simulink model "MCC_FUZZY"  (R2024a)
settings: Solver=VariableStepAuto  StartTime=0.0  StopTime=100.0  RelTol=1e-3
model workspace (MAT data in the model file):
  J = Simulink.Parameter
  J.Complexity = 'real'
  J.Dimensions = [0 0]
  J.DataType = 'auto'
  K = Simulink.Parameter
  K.Complexity = 'real'
  K.Dimensions = [0 0]
  K.DataType = 'auto'
  Kh = Simulink.Parameter
  Kh.Complexity = 'real'
  Kh.Dimensions = [0 0]
  Kh.DataType = 'auto'
  L = Simulink.Parameter
  L.Complexity = 'real'
  L.Dimensions = [0 0]
  L.DataType = 'auto'
  R = Simulink.Parameter
  R.Complexity = 'real'
  R.Dimensions = [0 0]
  R.DataType = 'auto'
  f = Simulink.Parameter
  f.Complexity = 'real'
  f.Dimensions = [0 0]
  f.DataType = 'auto'
libraries: fuzblock x1
settings Model: Creator=NB  LastModifiedBy=NB

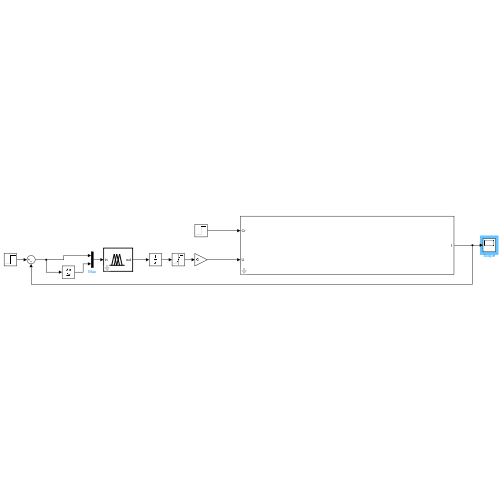
[thumbnail: Simulink's stored preview of the top-level diagram]
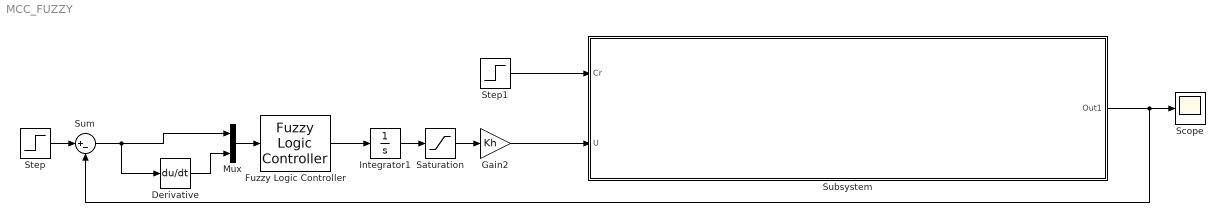
== system MCC_FUZZY ==
  Derivative : Derivative
  Fuzzy Logic Controller : fuzblock/Fuzzy Logic  Controller  FIS=FuzzyMCC  OutputSampleNumber=101  DataType=double  FuzzifiedInputs=off  RuleFiringStrengths=off  RuleOutputs=off  AggregatedOutputs=off  SimulateUsing=Interpreted execution  OutOfRangeInputValueMessage=warning  NoRuleFiredMessage=warning  EmptyOutputFuzzySetMessage=warning
  Gain2 : Gain  Gain=Kh  mask{Kh=1}
      mask prompts: Kh "entre Kh"
  Integrator1 : Integrator
  Mux : Mux  Inputs=2
  Saturation : Saturate  UpperLimit=220  LowerLimit=0
  Scope : Scope
  Step : Step  Time=0  After=100  SampleTime=0
  Step1 : Step  Time=50  After=0.05  SampleTime=0
  Subsystem : Subsystem  mask{R=2, L=0.1, J=0.05, f=0.01, K=0.01}
  Sum : Sum  Inputs=|+-
  wires:
  Subsystem/1(Out1) -> Sum/2, Scope/1
  Step1/1 -> Subsystem/1(Cr)
  Gain2/1 -> Subsystem/2(U)
  Step/1 -> Sum/1
  Fuzzy Logic Controller/1 -> Integrator1/1
  Mux/1 -> Fuzzy Logic Controller/1
  Derivative/1 -> Mux/2
  Sum/1 -> Derivative/1, Mux/1
  Integrator1/1 -> Saturation/1
  Saturation/1 -> Gain2/1

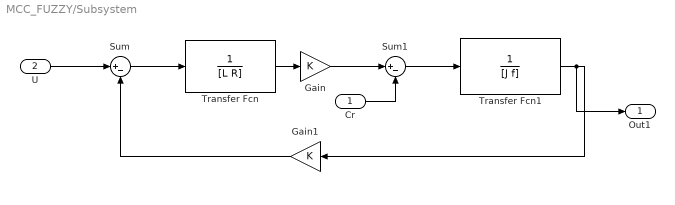
== system MCC_FUZZY/Subsystem ==
  Cr : Inport
  U : Inport  Port=2
  Gain : Gain  Gain=K
  Gain1 : Gain  Gain=K
  Sum : Sum  Inputs=|+-
  Sum1 : Sum  Inputs=|+-
  Transfer Fcn : TransferFcn  Denominator=[L R]
  Transfer Fcn1 : TransferFcn  Denominator=[J f]
  Out1 : Outport
  wires:
  Transfer Fcn/1 -> Gain/1
  Cr/1 -> Sum1/2
  Gain1/1 -> Sum/2
  U/1 -> Sum/1
  Gain/1 -> Sum1/1
  Transfer Fcn1/1 -> Out1/1, Gain1/1
  Sum/1 -> Transfer Fcn/1
  Sum1/1 -> Transfer Fcn1/1
